simulink subsystem "Controller"  (R2024b)
settings: Solver=VariableStepAuto  StartTime=0.0  StopTime=10.0  RelTol=1e-3
undefined symbols (not defined in the file or in its folder): flight_mode, Parameters, References
libraries: sharedtransform x13, eeGeneralControl x10, simulink x5, aerolibutil x2
(part 2 of 3)

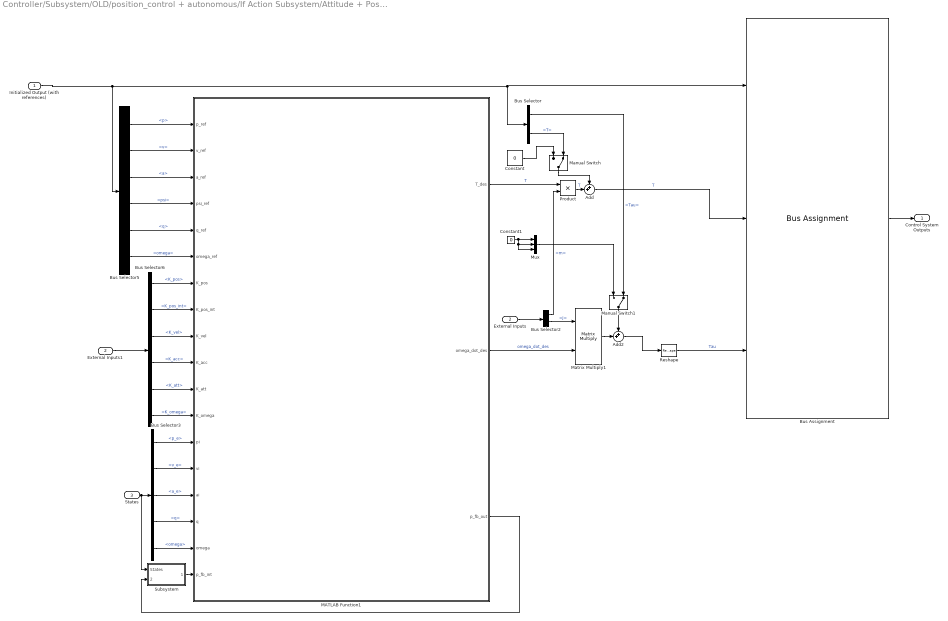
== system Controller/Subsystem/OLD/position_control + autonomous/If Action Subsystem/Attitude + Position FF control1 ==
  Initialized Output (with references) : Inport
  External Inputs : Inport  Port=2
  States : Inport  Port=3
  Add : Sum  Inputs=++|
  Add2 : Sum  Inputs=++|
  Bus Assignment : BusAssignment  AssignedSignals=Control Outputs.T,Control Outputs.Tau
  Bus Selector : BusSelector  OutputSignals=References.reconstructed.Tau,References.reconstructed.T
  Bus Selector2 : BusSelector  OutputSignals=Vehicle Parameters.m,Vehicle Parameters.J
  Bus Selector3 : BusSelector  OutputSignals=p_e,v_e,a_e,q,omega
  Bus Selector5 : BusSelector  OutputSignals=References.trajectory.p,References.trajectory.v,References.trajectory.a,References.trajectory.psi,References.reconstructed.q,References.reconstructed.omega
  Bus Selector6 : BusSelector  OutputSignals=Control Gains.K_pos,Control Gains.K_pos_int,Control Gains.K_vel,Control Gains.K_acc,Control Gains.K_att,Control Gains.K_omega
  Constant : Constant  Value=0
  Constant1 : Constant  Value=0
  External Inputs1 : InportShadow  Port=2
  MATLAB Function1 : MATLAB Function  TreatAsAtomicUnit=on
  Manual Switch : ManualSwitch  CurrentSetting=0
  Manual Switch1 : ManualSwitch  CurrentSetting=0
  Matrix Multiply1 : Product  Multiplication=Matrix(*)
  Mux : Mux  Inputs=3
  Product : Product
  Reshape : Reshape  OutputDimensionality=Column vector (2-D)
  Subsystem : Subsystem
  Control System Outputs : Outport
  wires:
  Manual Switch1/1 -> Add2/1
  Mux/1 -> Manual Switch1/1
  Constant1/1 -> Mux/1, Mux/2, Mux/3
  Constant/1 -> Manual Switch/1
  Manual Switch/1 -> Add/1
  Subsystem/1(p_fb_int) -> MATLAB Function1/18(p_fb_int)
  MATLAB Function1/3(p_fb_out) -> Subsystem/2(p_fb_out)
  Bus Selector6/2 -> MATLAB Function1/8(K_pos_int)  "<K_pos_int>"
  MATLAB Function1/2(omega_dot_des) -> Matrix Multiply1/2  "omega_dot_des"
  Bus Selector6/6 -> MATLAB Function1/12(K_omega)  "<K_omega>"
  Bus Selector6/5 -> MATLAB Function1/11(K_att)  "<K_att>"
  Initialized Output (with references)/1 -> Bus Assignment/1, Bus Selector/1, Bus Selector5/1
  Bus Selector5/4 -> MATLAB Function1/4(psi_ref)  "<psi>"
  Bus Selector6/4 -> MATLAB Function1/10(K_acc)  "<K_acc>"
  Bus Selector6/3 -> MATLAB Function1/9(K_vel)  "<K_vel>"
  Bus Selector6/1 -> MATLAB Function1/7(K_pos)  "<K_pos>"
  External Inputs1/1 -> Bus Selector6/1
  Bus Selector2/2 -> Matrix Multiply1/1  "<J>"
  External Inputs/1 -> Bus Selector2/1
  Matrix Multiply1/1 -> Add2/2
  Add2/1 -> Reshape/1
  Bus Selector/1 -> Manual Switch1/2  "<Tau>"
  Bus Selector/2 -> Manual Switch/2  "<T>"
  Bus Selector3/3 -> MATLAB Function1/15(ai)  "<a_e>"
  Bus Selector3/2 -> MATLAB Function1/14(vi)  "<v_e>"
  Bus Selector3/5 -> MATLAB Function1/17(omega)  "<omega>"
  Bus Selector3/4 -> MATLAB Function1/16(q)  "<q>"
  Bus Selector3/1 -> MATLAB Function1/13(pi)  "<p_e>"
  States/1 -> Bus Selector3/1, Subsystem/1(States)
  Bus Selector5/6 -> MATLAB Function1/6(omega_ref)  "<omega>"
  Bus Selector5/5 -> MATLAB Function1/5(q_ref)  "<q>"
  Bus Selector5/3 -> MATLAB Function1/3(a_ref)  "<a>"
  Bus Selector5/2 -> MATLAB Function1/2(v_ref)  "<v>"
  Bus Selector5/1 -> MATLAB Function1/1(p_ref)  "<p>"
  Bus Assignment/1 -> Control System Outputs/1
  Reshape/1 -> Bus Assignment/3  "Tau"
  Add/1 -> Bus Assignment/2  "T"
  Bus Selector2/1 -> Product/2  "<m>"
  MATLAB Function1/1(T_des) -> Product/1  "T"
  Product/1 -> Add/2  "T"

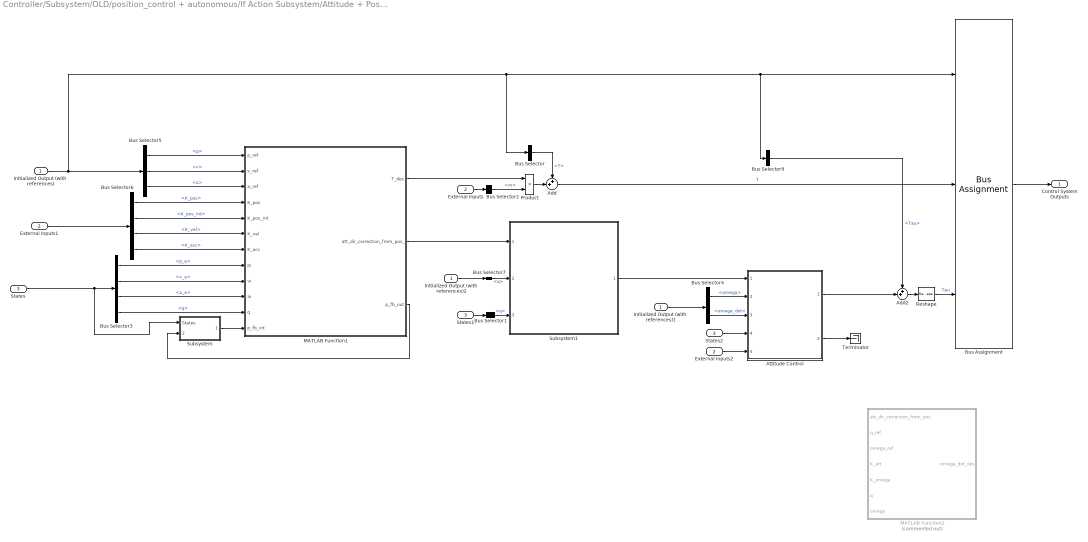
== system Controller/Subsystem/OLD/position_control + autonomous/If Action Subsystem/Attitude + Position FF control2 ==
  Initialized Output (with references) : Inport
  External Inputs : Inport  Port=2
  States : Inport  Port=3
  Add : Sum  Inputs=++|
  Add2 : Sum  Inputs=++|
  Attitude Control : Subsystem  ReferencedSubsystem=Attitude_Control
  Bus Assignment : BusAssignment  AssignedSignals=Control Outputs.T,Control Outputs.Tau
  Bus Selector : BusSelector  OutputSignals=References.reconstructed.T
  Bus Selector1 : BusSelector  OutputSignals=q
  Bus Selector2 : BusSelector  OutputSignals=Vehicle Parameters.m
  Bus Selector3 : BusSelector  OutputSignals=p_e,v_e,a_e,q
  Bus Selector4 : BusSelector  OutputSignals=References.reconstructed.omega,References.reconstructed.omega_dot
  Bus Selector5 : BusSelector  OutputSignals=References.trajectory.p,References.trajectory.v,References.trajectory.a
  Bus Selector6 : BusSelector  OutputSignals=Control Gains.K_pos,Control Gains.K_pos_int,Control Gains.K_vel,Control Gains.K_acc
  Bus Selector7 : BusSelector  OutputSignals=References.reconstructed.q
  Bus Selector9 : BusSelector  OutputSignals=References.reconstructed.Tau
  External Inputs1 : InportShadow  Port=2
  External Inputs2 : InportShadow  Port=2
  Initialized Output (with references)1 : InportShadow
  Initialized Output (with references)2 : InportShadow
  MATLAB Function1 : MATLAB Function  TreatAsAtomicUnit=on
  MATLAB Function2 : MATLAB Function  Commented=on  TreatAsAtomicUnit=on
  Product : Product
  Reshape : Reshape  OutputDimensionality=Column vector (2-D)
  States1 : InportShadow  Port=3
  States2 : InportShadow  Port=3
  Subsystem : Subsystem
  Subsystem1 : Subsystem  ReferencedSubsystem=CombineOuterLoopFB_with_FF_att_ref
  Terminator : Terminator
  Control System Outputs : Outport
  wires:
  Bus Selector9/1 -> Add2/1  "<Tau>"
  Subsystem/1(p_fb_int) -> MATLAB Function1/12(p_fb_int)
  MATLAB Function1/3(p_fb_out) -> Subsystem/2(p_fb_out)
  Bus Selector6/2 -> MATLAB Function1/5(K_pos_int)  "<K_pos_int>"
  Bus Selector6/4 -> MATLAB Function1/7(K_acc)  "<K_acc>"
  Bus Selector6/3 -> MATLAB Function1/6(K_vel)  "<K_vel>"
  Bus Selector6/1 -> MATLAB Function1/4(K_pos)  "<K_pos>"
  Attitude Control/1 -> Add2/2
  Add2/1 -> Reshape/1
  Bus Selector/1 -> Add/1  "<T>"
  Bus Selector3/3 -> MATLAB Function1/10(ai)  "<a_e>"
  Bus Selector3/2 -> MATLAB Function1/9(vi)  "<v_e>"
  Bus Selector3/4 -> MATLAB Function1/11(q)  "<q>"
  Bus Selector3/1 -> MATLAB Function1/8(pi)  "<p_e>"
  Bus Selector5/3 -> MATLAB Function1/3(a_ref)  "<a>"
  Bus Selector5/2 -> MATLAB Function1/2(v_ref)  "<v>"
  Bus Selector5/1 -> MATLAB Function1/1(p_ref)  "<p>"
  Bus Assignment/1 -> Control System Outputs/1
  Reshape/1 -> Bus Assignment/3  "Tau"
  Add/1 -> Bus Assignment/2  "T"
  Bus Selector2/1 -> Product/2  "<m>"
  Bus Selector4/1 -> Attitude Control/2  "<omega>"
  Initialized Output (with references)/1 -> Bus Selector5/1, Bus Selector/1, Bus Selector9/1, Bus Assignment/1
  External Inputs1/1 -> Bus Selector6/1
  States/1 -> Subsystem/1(States), Bus Selector3/1
  Product/1 -> Add/2
  MATLAB Function1/2(att_dir_correction_from_pos_) -> Subsystem1/1
  MATLAB Function1/1(T_des) -> Product/1
  External Inputs/1 -> Bus Selector2/1
  Initialized Output (with references)1/1 -> Bus Selector4/1
  Bus Selector4/2 -> Attitude Control/3  "<omega_dot>"
  Attitude Control/2 -> Terminator/1
  Subsystem1/1 -> Attitude Control/1
  External Inputs2/1 -> Attitude Control/5
  States2/1 -> Attitude Control/4
  Initialized Output (with references)2/1 -> Bus Selector7/1
  States1/1 -> Bus Selector1/1
  Bus Selector1/1 -> Subsystem1/3  "<q>"
  Bus Selector7/1 -> Subsystem1/2  "<q>"

== system Controller/Subsystem/OLD/position_control + autonomous/K-matrix control/K-matrix-control ==
  Initialized Output (with references) : Inport
  External Inputs : Inport  Port=2
  States : Inport  Port=3
  Bus Assignment : BusAssignment  AssignedSignals=Control Outputs.Tau,Control Outputs.T
  Bus Selector : BusSelector  OutputSignals=References.trajectory.p,References.trajectory.v,References.reconstructed.q,References.reconstructed.omega,References.reconstructed.T,References.reconstructed.Tau
  Bus Selector1 : BusSelector  OutputSignals=Control Gains.K_matrix_control.K_pos_int
  Bus Selector3 : BusSelector  OutputSignals=p_e,v_e,q,omega_b
  Bus Selector4 : BusSelector  OutputSignals=Control Gains.K_matrix_control.K
  External Inputs1 : InportShadow  Port=2
  MATLAB Function2 : MATLAB Function  TreatAsAtomicUnit=on
  Product : Product  Multiplication=Matrix(*)
  Reshape : Reshape  OutputDimensionality=Column vector (2-D)
  States1 : InportShadow  Port=3
  Subsystem : Subsystem
  Subsystem3 : Subsystem
  Control System Outputs : Outport
  wires:
  Subsystem/1(att) -> MATLAB Function2/8(att_ref)
  Bus Selector/3 -> Subsystem/1(q)  "<q>"
  Bus Selector/4 -> MATLAB Function2/9(w_ref)  "<omega>"
  Bus Selector/5 -> MATLAB Function2/10(T_ref)  "<T>"
  Bus Selector/6 -> MATLAB Function2/11(Tau_ref)  "<Tau>"
  Bus Selector4/1 -> MATLAB Function2/5(K)  "<K>"
  States/1 -> Bus Selector3/1
  Bus Selector3/4 -> MATLAB Function2/4(omega)  "<omega_b>"
  Bus Selector3/3 -> MATLAB Function2/3(q)  "<q>"
  External Inputs/1 -> Bus Selector4/1
  MATLAB Function2/2(T_des) -> Bus Assignment/3  "T"
  Reshape/1 -> Bus Assignment/2  "Tau"
  MATLAB Function2/1(Tau_des) -> Reshape/1
  Initialized Output (with references)/1 -> Bus Assignment/1, Bus Selector/1
  Bus Assignment/1 -> Control System Outputs/1
  States1/1 -> Subsystem3/1(States)
  Subsystem3/1(p_fb_int) -> Product/2
  MATLAB Function2/3(p_fb_out) -> Subsystem3/2(p_fb_out)
  External Inputs1/1 -> Bus Selector1/1
  Bus Selector1/1 -> Product/1  "<K_pos_int>"
  Bus Selector/2 -> MATLAB Function2/7(V_ref)  "<v>"
  Bus Selector/1 -> MATLAB Function2/6(R_ref)  "<p>"
  Bus Selector3/1 -> MATLAB Function2/1(pi)  "<p_e>"
  Bus Selector3/2 -> MATLAB Function2/2(vi)  "<v_e>"
  Product/1 -> MATLAB Function2/12(p_fb_int)

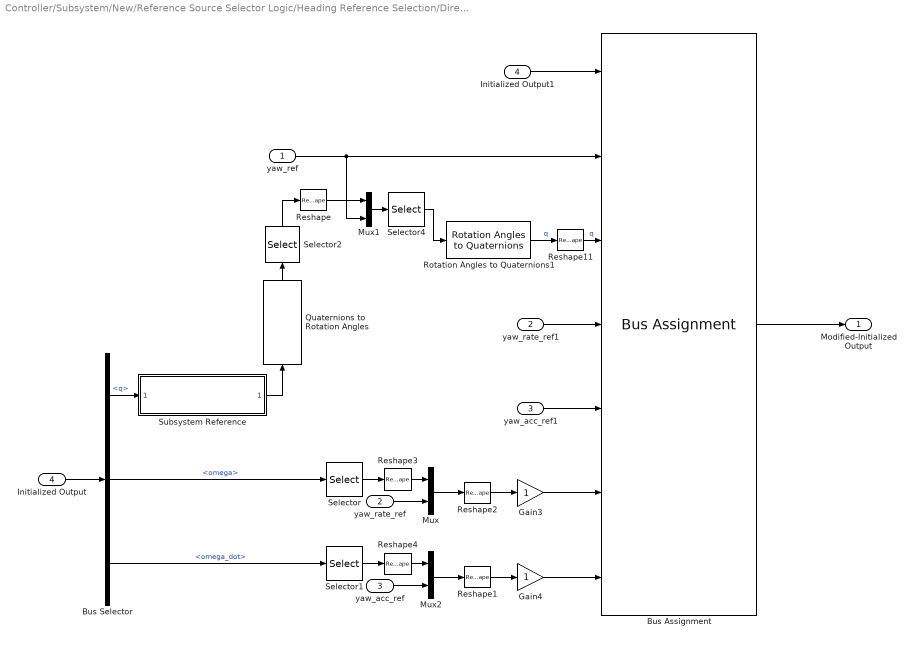
== system Controller/Subsystem/New/Reference Source Selector Logic/Heading Reference Selection/Direct Yaw Command/Subsystem ==
  yaw_ref : Inport
  yaw_rate_ref : Inport  Port=2
  yaw_acc_ref : Inport  Port=3
  Initialized Output : Inport  Port=4
  Bus Assignment : BusAssignment  AssignedSignals=References.trajectory.psi,References.reconstructed.q,References.trajectory.psi_dot,References.trajectory.psi_ddot,References.reconstructed.omega,References.reconstructed.omega_dot
  Bus Selector : BusSelector  OutputSignals=References.reconstructed.q,References.reconstructed.omega,References.reconstructed.omega_dot
  Gain3 : Gain
  Gain4 : Gain
  Initialized Output1 : InportShadow  Port=4
  Mux : Mux  Inputs=2
  Mux1 : Mux  Inputs=2
  Mux2 : Mux  Inputs=2
  Quaternions to Rotation Angles : sharedtransform/Quaternions to Rotation Angles  rotationOrder=ZYX  aMode=aMode
  Reshape : Reshape
  Reshape1 : Reshape  OutputDimensionality=Column vector (2-D)
  Reshape11 : Reshape  OutputDimensionality=Row vector (2-D)
  Reshape2 : Reshape  OutputDimensionality=Column vector (2-D)
  Reshape3 : Reshape
  Reshape4 : Reshape
  Rotation Angles to Quaternions1 : sharedtransform/Rotation Angles to Quaternions  rotationOrder=ZYX  aMode=aMode
  Selector : Selector  InputPortWidth=3  IndexOptions=Index vector (dialog)  Indices=[1 2]  OutputSizes=1
  Selector1 : Selector  InputPortWidth=3  IndexOptions=Index vector (dialog)  Indices=[1 2]  OutputSizes=1
  Selector2 : Selector  InputPortWidth=3  IndexOptions=Index vector (dialog)  Indices=[3 2]  OutputSizes=1
  Selector4 : Selector  InputPortWidth=3  IndexOptions=Index vector (dialog)  Indices=[3 2 1]  OutputSizes=1
  Subsystem Reference : Subsystem  ReferencedSubsystem=Check_Quat
  yaw_acc_ref1 : InportShadow  Port=3
  yaw_rate_ref1 : InportShadow  Port=2
  Modified-Initialized Output : Outport
  wires:
  Bus Assignment/1 -> Modified-Initialized Output/1
  yaw_acc_ref/1 -> Mux2/2
  Gain4/1 -> Bus Assignment/7
  Gain3/1 -> Bus Assignment/6
  yaw_rate_ref/1 -> Mux/2
  Reshape1/1 -> Gain4/1
  Reshape2/1 -> Gain3/1
  Bus Selector/3 -> Selector1/1  "<omega_dot>"
  Selector/1 -> Reshape3/1
  Reshape3/1 -> Mux/1
  Mux/1 -> Reshape2/1
  Selector1/1 -> Reshape4/1
  Reshape4/1 -> Mux2/1
  Mux2/1 -> Reshape1/1
  Initialized Output/1 -> Bus Selector/1
  Bus Selector/2 -> Selector/1  "<omega>"
  Bus Selector/1 -> Subsystem Reference/1  "<q>"
  yaw_ref/1 -> Mux1/2, Bus Assignment/2
  Quaternions to Rotation Angles/1 -> Selector2/1
  Selector2/1 -> Reshape/1
  Reshape/1 -> Mux1/1
  Rotation Angles to Quaternions1/1 -> Reshape11/1  "q"
  Reshape11/1 -> Bus Assignment/3  "q"
  Mux1/1 -> Selector4/1
  Selector4/1 -> Rotation Angles to Quaternions1/1
  yaw_rate_ref1/1 -> Bus Assignment/4
  yaw_acc_ref1/1 -> Bus Assignment/5
  Initialized Output1/1 -> Bus Assignment/1
  Subsystem Reference/1 -> Quaternions to Rotation Angles/1

== system Controller/Subsystem/New/Reference Source Selector Logic/Thrust Reference Selection/Direct Thrust Command/Subsystem1 ==
  T : Inport
  Initialized Output : Inport  Port=2
  Bus Assignment : BusAssignment  AssignedSignals=References.reconstructed.T,Control Outputs.T
  Control Outputs : Outport
  wires:
  Bus Assignment/1 -> Control Outputs/1
  Initialized Output/1 -> Bus Assignment/1
  T/1 -> Bus Assignment/3, Bus Assignment/2  "T"

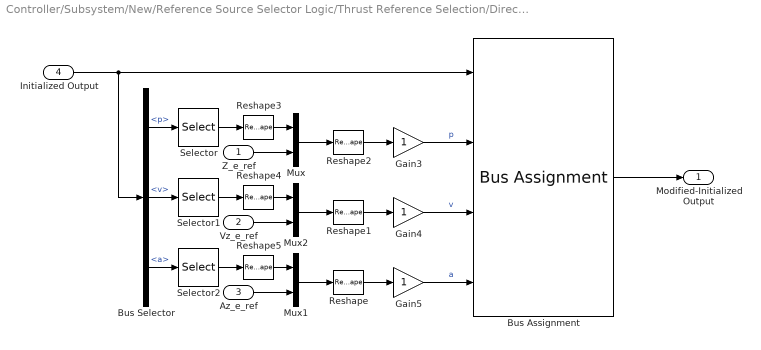
== system Controller/Subsystem/New/Reference Source Selector Logic/Thrust Reference Selection/Direct Z Position Command/Subsystem ==
  Z_e_ref : Inport
  Vz_e_ref : Inport  Port=2
  Az_e_ref : Inport  Port=3
  Initialized Output : Inport  Port=4
  Bus Assignment : BusAssignment  AssignedSignals=References.trajectory.p,References.trajectory.v,References.trajectory.a
  Bus Selector : BusSelector  OutputSignals=References.trajectory.p,References.trajectory.v,References.trajectory.a
  Gain3 : Gain
  Gain4 : Gain
  Gain5 : Gain
  Mux : Mux  Inputs=2
  Mux1 : Mux  Inputs=2
  Mux2 : Mux  Inputs=2
  Reshape : Reshape  OutputDimensionality=Column vector (2-D)
  Reshape1 : Reshape  OutputDimensionality=Column vector (2-D)
  Reshape2 : Reshape  OutputDimensionality=Column vector (2-D)
  Reshape3 : Reshape
  Reshape4 : Reshape
  Reshape5 : Reshape
  Selector : Selector  InputPortWidth=3  IndexOptions=Index vector (dialog)  Indices=[1 2]  OutputSizes=1
  Selector1 : Selector  InputPortWidth=3  IndexOptions=Index vector (dialog)  Indices=[1 2]  OutputSizes=1
  Selector2 : Selector  InputPortWidth=3  IndexOptions=Index vector (dialog)  Indices=[1 2]  OutputSizes=1
  Modified-Initialized Output : Outport
  wires:
  Bus Assignment/1 -> Modified-Initialized Output/1
  Vz_e_ref/1 -> Mux2/2
  Gain4/1 -> Bus Assignment/3  "v"
  Gain5/1 -> Bus Assignment/4  "a"
  Gain3/1 -> Bus Assignment/2  "p"
  Z_e_ref/1 -> Mux/2
  Reshape/1 -> Gain5/1
  Reshape1/1 -> Gain4/1
  Reshape2/1 -> Gain3/1
  Bus Selector/1 -> Selector/1  "<p>"
  Bus Selector/2 -> Selector1/1  "<v>"
  Bus Selector/3 -> Selector2/1  "<a>"
  Selector/1 -> Reshape3/1
  Reshape3/1 -> Mux/1
  Mux/1 -> Reshape2/1
  Selector1/1 -> Reshape4/1
  Reshape4/1 -> Mux2/1
  Mux2/1 -> Reshape1/1
  Mux1/1 -> Reshape/1
  Reshape5/1 -> Mux1/1
  Selector2/1 -> Reshape5/1
  Az_e_ref/1 -> Mux1/2
  Initialized Output/1 -> Bus Selector/1, Bus Assignment/1

== system Controller/Subsystem/New/Reference Source Selector Logic/[X, Y] and//or [Roll, Pitch] Reference Selection/Direct Roll and Pitch Command/Subsystem1 ==
  Roll_Pitch_ref : Inport
  Roll_Pitch_Rate_ref : Inport  Port=2
  Roll_Pitch_Acc_ref : Inport  Port=3
  Initialized Output : Inport  Port=4
  Bus Assignment : BusAssignment  AssignedSignals=References.reconstructed.q,References.reconstructed.omega,References.reconstructed.omega_dot
  Bus Selector : BusSelector  OutputSignals=References.trajectory.psi,References.trajectory.psi_dot,References.trajectory.psi_ddot
  Mux : Mux  Inputs=2
  Mux1 : Mux  Inputs=2
  Mux2 : Mux  Inputs=2
  Reshape : Reshape
  Reshape1 : Reshape
  Reshape11 : Reshape  OutputDimensionality=Row vector (2-D)
  Reshape2 : Reshape
  Reshape7 : Reshape  OutputDimensionality=Column vector (2-D)
  Reshape8 : Reshape  OutputDimensionality=Column vector (2-D)
  Rotation Angles to Quaternions : sharedtransform/Rotation Angles to Quaternions  rotationOrder=ZYX  aMode=aMode
  Selector2 : Selector  InputPortWidth=3  IndexOptions=Index vector (dialog)  Indices=[3 2 1]  OutputSizes=1
  Control Outputs : Outport
  wires:
  Selector2/1 -> Rotation Angles to Quaternions/1
  Bus Assignment/1 -> Control Outputs/1
  Initialized Output/1 -> Bus Selector/1, Bus Assignment/1
  Mux2/1 -> Reshape8/1
  Reshape11/1 -> Bus Assignment/2  "q"
  Reshape8/1 -> Bus Assignment/4  "omega_dot"
  Rotation Angles to Quaternions/1 -> Reshape11/1  "q"
  Reshape7/1 -> Bus Assignment/3  "omega"
  Mux/1 -> Selector2/1
  Mux1/1 -> Reshape7/1
  Roll_Pitch_ref/1 -> Reshape/1
  Bus Selector/1 -> Mux/2  "<psi>"
  Reshape/1 -> Mux/1
  Roll_Pitch_Rate_ref/1 -> Reshape1/1
  Reshape1/1 -> Mux1/1
  Bus Selector/2 -> Mux1/2  "<psi_dot>"
  Bus Selector/3 -> Mux2/2  "<psi_ddot>"
  Reshape2/1 -> Mux2/1
  Roll_Pitch_Acc_ref/1 -> Reshape2/1

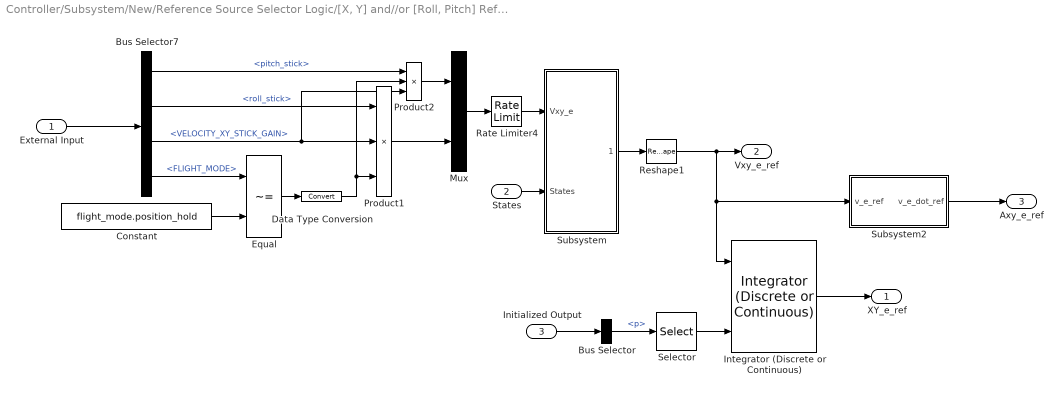
== system Controller/Subsystem/New/Reference Source Selector Logic/[X, Y] and//or [Roll, Pitch] Reference Selection/Direct XY Position Command /Direct XY Position Command  ==
  External Input : Inport
  States : Inport  Port=2
  Initialized Output : Inport  Port=3
  Bus Selector : BusSelector  OutputSignals=References.trajectory.p
  Bus Selector7 : BusSelector  OutputSignals=Pilot Input.Sticks.pitch_stick,Pilot Input.Sticks.roll_stick,Pilot Input.Parameters.VELOCITY_XY_STICK_GAIN,Pilot Input.FLIGHT_MODE
  Constant : Constant  Value=flight_mode.position_hold
  Data Type Conversion : DataTypeConversion  SaturateOnIntegerOverflow=off  RndMeth=Floor
  Equal : RelationalOperator  Operator=~=  OutDataTypeStr=boolean  RndMeth=Simplest  InputSameDT=off
  Integrator (Discrete or Continuous) : eeGeneralControl/Integrator (Discrete or Continuous)  LabelModeActiveChoice=Discrete  ExternalReset=either  LimitType=Anti-windup  B=inf  A=-inf  Ts=-1
      settings: LibrarySourceBlock=|
      | ee_sl_lib/General Control/Integrator
      | (Discrete or Continuous)
  Mux : Mux  Inputs=2
  Product1 : Product  Inputs=3
  Product2 : Product  Inputs=3
  Rate Limiter4 : RateLimiter  RisingSlewLimit=3  FallingSlewLimit=-3  SampleTimeMode=inherited
  Reshape1 : Reshape
  Selector : Selector  InputPortWidth=3  IndexOptions=Index vector (dialog)  Indices=[1 2]  OutputSizes=1
  Subsystem : Subsystem
  Subsystem2 : Subsystem
  XY_e_ref : Outport
  Vxy_e_ref : Outport  Port=2
  Axy_e_ref : Outport  Port=3
  wires:
  Subsystem/1("[Vx Vy]_b") -> Reshape1/1
  States/1 -> Subsystem/2(States)
  Bus Selector7/3 -> Product2/3, Product1/2  "<VELOCITY_XY_STICK_GAIN>"
  Product2/1 -> Mux/1
  Product1/1 -> Mux/2
  External Input/1 -> Bus Selector7/1
  Bus Selector7/1 -> Product2/1  "<pitch_stick>"
  Bus Selector7/2 -> Product1/1  "<roll_stick>"
  Rate Limiter4/1 -> Subsystem/1(Vxy_e)
  Reshape1/1 -> Subsystem2/1(v_e_ref), Integrator (Discrete or Continuous)/1, Vxy_e_ref/1
  Initialized Output/1 -> Bus Selector/1
  Bus Selector/1 -> Selector/1  "<p>"
  Subsystem2/1(v_e_dot_ref) -> Axy_e_ref/1
  Integrator (Discrete or Continuous)/1 -> XY_e_ref/1
  Selector/1 -> Integrator (Discrete or Continuous)/3
  Equal/1 -> Data Type Conversion/1
  Mux/1 -> Rate Limiter4/1
  Data Type Conversion/1 -> Product2/2, Product1/3
  Constant/1 -> Equal/2
  Bus Selector7/4 -> Equal/1  "<FLIGHT_MODE>"

== system Controller/Subsystem/New/Reference Source Selector Logic/[X, Y] and//or [Roll, Pitch] Reference Selection/Direct XY Position Command /Subsystem1 ==
  XY_e_ref : Inport
  Vxy_e_ref : Inport  Port=2
  Axy_e_ref : Inport  Port=3
  Initialized Output : Inport  Port=4
  Bus Assignment : BusAssignment  AssignedSignals=References.trajectory.p,References.trajectory.v,References.trajectory.a
  Bus Selector : BusSelector  OutputSignals=References.trajectory.p,References.trajectory.v,References.trajectory.a
  Mux : Mux  Inputs=2
  Mux1 : Mux  Inputs=2
  Mux2 : Mux  Inputs=2
  Reshape : Reshape
  Reshape1 : Reshape
  Reshape2 : Reshape
  Reshape3 : Reshape  OutputDimensionality=Column vector (2-D)
  Reshape7 : Reshape  OutputDimensionality=Column vector (2-D)
  Reshape8 : Reshape  OutputDimensionality=Column vector (2-D)
  Selector : Selector  InputPortWidth=3  IndexOptions=Index vector (dialog)  Indices=[3]  OutputSizes=1
  Selector1 : Selector  InputPortWidth=3  IndexOptions=Index vector (dialog)  Indices=[3]  OutputSizes=1
  Selector2 : Selector  InputPortWidth=3  IndexOptions=Index vector (dialog)  Indices=[3]  OutputSizes=1
  Control Outputs : Outport
  wires:
  Bus Assignment/1 -> Control Outputs/1
  Initialized Output/1 -> Bus Selector/1, Bus Assignment/1
  Mux2/1 -> Reshape8/1
  Reshape3/1 -> Bus Assignment/2  "p_e"
  Reshape8/1 -> Bus Assignment/4  "a_e"
  Reshape7/1 -> Bus Assignment/3  "v_e"
  Mux/1 -> Reshape3/1
  Mux1/1 -> Reshape7/1
  XY_e_ref/1 -> Reshape/1
  Bus Selector/1 -> Selector2/1  "<p>"
  Reshape/1 -> Mux/1
  Vxy_e_ref/1 -> Reshape1/1
  Reshape1/1 -> Mux1/1
  Bus Selector/2 -> Selector1/1  "<v>"
  Bus Selector/3 -> Selector/1  "<a>"
  Reshape2/1 -> Mux2/1
  Axy_e_ref/1 -> Reshape2/1
  Selector/1 -> Mux2/2
  Selector1/1 -> Mux1/2
  Selector2/1 -> Mux/2

== system Controller/Subsystem/New/Translational Motion Feedback Selector/Switch Case Action Subsystem/Translational Motion Control/Subsystem ==
  <MIN_TH> : Inport
  <MAX_TH> : Inport  Port=2
  <MAX_THRUST> : Inport  Port=3
  Gain : Gain  Gain=4
  Product : Product
  Product1 : Product
  MIN_TH : Outport
  MAX_TH : Outport  Port=2
  wires:
  Gain/1 -> Product/1, Product1/2
  <MAX_TH>/1 -> Product1/1
  <MIN_TH>/1 -> Product/2
  Product/1 -> MIN_TH/1
  Product1/1 -> MAX_TH/1
  <MAX_THRUST>/1 -> Gain/1

== system Controller/Subsystem/OLD/position_control + autonomous/Guidance/Trajectory Solution Evaluator/Hold current position ==
  Initialized Output : Inport
  Action Port : ActionPort  InitializeStates=reset
  Subsystem1 : Subsystem
  Modified-Initialized Output : Outport
  wires:
  Initialized Output/1 -> Subsystem1/1(Initialized Output)
  Subsystem1/1(Modified-Initialized Output) -> Modified-Initialized Output/1

== system Controller/Subsystem/OLD/position_control + autonomous/Guidance/Trajectory Solution Evaluator/Switch Case Action Subsystem ==
  external_input : Inport
  States : Inport  Port=2
  Initialized Output : Inport  Port=3
  Action Port : ActionPort  InitializeStates=reset
  FF reconstructor : Subsystem  ReferencedSubsystem=FF_reconstructor
  Modified-Initialized Output : Outport
  wires:
  external_input/1 -> FF reconstructor/2
  States/1 -> FF reconstructor/3
  FF reconstructor/1 -> Modified-Initialized Output/1
  Initialized Output/1 -> FF reconstructor/1

== system Controller/Subsystem/OLD/position_control + autonomous/Guidance/Trajectory Solution Evaluator/Switch Case Action Subsystem1 ==
  States : Inport
  external_input : Inport  Port=2
  Initialized Output : Inport  Port=3
  Action Port : ActionPort  InitializeStates=reset
  Constant : Constant  Value=false
  Delay : Delay  DelayLength=1  InitialCondition=true
  Map User Input : Subsystem
  Modified-Initialized Output : Outport
  wires:
  Delay/1 -> Map User Input/4(reset)
  Constant/1 -> Delay/1
  Initialized Output/1 -> Map User Input/3(Initialized Output)
  Map User Input/1(Modified-Initialized Output) -> Modified-Initialized Output/1
  external_input/1 -> Map User Input/1(External Input)
  States/1 -> Map User Input/2(States)

== system Controller/Subsystem/OLD/position_control + autonomous/If Action Subsystem/Attitude + Position FF control/Subsystem ==
  States : Inport
  p_fb_out : Inport  Port=2
  Bus Selector1 : BusSelector  OutputSignals=GC
  If : If  IfExpression=u1
  If Action Subsystem : Subsystem  TreatAsAtomicUnit=on
  If Action Subsystem1 : Subsystem  TreatAsAtomicUnit=on
  Merge : Merge
  p_fb_int : Outport
  wires:
  Merge/1 -> p_fb_int/1
  If Action Subsystem1/1(Out1) -> Merge/2
  If Action Subsystem/1(p_fb_int) -> Merge/1
  If/2 -> If Action Subsystem/Action
  States/1 -> Bus Selector1/1
  p_fb_out/1 -> If Action Subsystem/1(p_fb_out)
  If/1 -> If Action Subsystem1/Action
  Bus Selector1/1 -> If/1  "<GC>"

== system Controller/Subsystem/OLD/position_control + autonomous/If Action Subsystem/Attitude + Position FF control1/Subsystem ==
  States : Inport
  p_fb_out : Inport  Port=2
  Bus Selector1 : BusSelector  OutputSignals=GC
  If : If  IfExpression=u1
  If Action Subsystem : Subsystem  TreatAsAtomicUnit=on
  If Action Subsystem1 : Subsystem  TreatAsAtomicUnit=on
  Merge : Merge
  p_fb_int : Outport
  wires:
  Merge/1 -> p_fb_int/1
  If Action Subsystem1/1(Out1) -> Merge/2
  If Action Subsystem/1(p_fb_int) -> Merge/1
  If/2 -> If Action Subsystem/Action
  States/1 -> Bus Selector1/1
  p_fb_out/1 -> If Action Subsystem/1(p_fb_out)
  If/1 -> If Action Subsystem1/Action
  Bus Selector1/1 -> If/1  "<GC>"

== system Controller/Subsystem/OLD/position_control + autonomous/If Action Subsystem/Attitude + Position FF control2/Subsystem ==
  States : Inport
  p_fb_out : Inport  Port=2
  Bus Selector1 : BusSelector  OutputSignals=GC
  If : If  IfExpression=u1
  If Action Subsystem : Subsystem  TreatAsAtomicUnit=on
  If Action Subsystem1 : Subsystem  TreatAsAtomicUnit=on
  Merge : Merge
  p_fb_int : Outport
  wires:
  Merge/1 -> p_fb_int/1
  If Action Subsystem1/1(Out1) -> Merge/2
  If Action Subsystem/1(p_fb_int) -> Merge/1
  If/2 -> If Action Subsystem/Action
  States/1 -> Bus Selector1/1
  p_fb_out/1 -> If Action Subsystem/1(p_fb_out)
  If/1 -> If Action Subsystem1/Action
  Bus Selector1/1 -> If/1  "<GC>"

== system Controller/Subsystem/OLD/position_control + autonomous/K-matrix control/K-matrix-control/Subsystem ==
  q : Inport
  Quaternions to Rotation Angles : sharedtransform/Quaternions to Rotation Angles  rotationOrder=ZYX  aMode=aMode
  Reshape1 : Reshape  OutputDimensionality=Column vector (2-D)
  Selector : Selector  InputPortWidth=3  IndexOptions=Index vector (dialog)  Indices=[3 2 1]  OutputSizes=1
  att : Outport
  wires:
  Reshape1/1 -> att/1
  q/1 -> Quaternions to Rotation Angles/1
  Quaternions to Rotation Angles/1 -> Selector/1
  Selector/1 -> Reshape1/1

== system Controller/Subsystem/OLD/position_control + autonomous/K-matrix control/K-matrix-control/Subsystem3 ==
  States : Inport
  p_fb_out : Inport  Port=2
  Bus Selector1 : BusSelector  OutputSignals=GC
  If : If  IfExpression=u1
  If Action Subsystem : Subsystem  TreatAsAtomicUnit=on
  If Action Subsystem1 : Subsystem  TreatAsAtomicUnit=on
  Merge : Merge
  p_fb_int : Outport
  wires:
  Merge/1 -> p_fb_int/1
  If Action Subsystem1/1(Out1) -> Merge/2
  If Action Subsystem/1(p_fb_int) -> Merge/1
  If/2 -> If Action Subsystem/Action
  States/1 -> Bus Selector1/1
  p_fb_out/1 -> If Action Subsystem/1(p_fb_out)
  If/1 -> If Action Subsystem1/Action
  Bus Selector1/1 -> If/1  "<GC>"

== system Controller/Subsystem/New/Reference Source Selector Logic/[X, Y] and//or [Roll, Pitch] Reference Selection/Direct XY Position Command /Direct XY Position Command /Subsystem ==
  Vxy_e : Inport
  States : Inport  Port=2
  Bus Selector1 : BusSelector  OutputSignals=att
  Constant : Constant  Value=0
  Gain : Gain  Gain=-1
  Mux1 : Mux  Inputs=3
  Mux2 : Mux  Inputs=2
  Quaternion Rotation : aerolibutil/Quaternion Rotation
  Rotation Angles to Quaternions : sharedtransform/Rotation Angles to Quaternions  rotationOrder=ZYX  aMode=aMode
  Selector : Selector  InputPortWidth=3  IndexOptions=Index vector (dialog)  Indices=[3]  OutputSizes=1
  Selector1 : Selector  InputPortWidth=3  IndexOptions=Index vector (dialog)  Indices=[1,2]  OutputSizes=1
  "[Vx Vy]_b" : Outport
  wires:
  Gain/1 -> Mux1/1
  Vxy_e/1 -> Mux2/1
  Rotation Angles to Quaternions/1 -> Quaternion Rotation/1
  Bus Selector1/1 -> Selector/1  "<att>"
  Selector/1 -> Gain/1
  Quaternion Rotation/1 -> Selector1/1
  Constant/1 -> Mux1/2, Mux2/2, Mux1/3
  Mux2/1 -> Quaternion Rotation/2
  States/1 -> Bus Selector1/1
  Mux1/1 -> Rotation Angles to Quaternions/1
  Selector1/1 -> "[Vx Vy]_b"/1

== system Controller/Subsystem/New/Reference Source Selector Logic/[X, Y] and//or [Roll, Pitch] Reference Selection/Direct XY Position Command /Direct XY Position Command /Subsystem2 ==
  v_e_ref : Inport
  Discrete Derivative : simulink/Discrete/Discrete Derivative  gainval=1.0  ICPrevScaledInput=0.0  OutMin=[]  OutMax=[]  OutDataType=fixdt(1, 16)  OutScaling=2^-10  DoSatur=off
  Low-Pass Filter (Discrete or Continuous) : eeGeneralControl/Low-Pass Filter (Discrete or Continuous)  K=1  T=1/40  B=inf  A=-inf  init_option=Inherited from block input  x0=0  Ts=-1
  v_e_dot_ref : Outport
  wires:
  Low-Pass Filter (Discrete or Continuous)/1 -> v_e_dot_ref/1
  v_e_ref/1 -> Discrete Derivative/1
  Discrete Derivative/1 -> Low-Pass Filter (Discrete or Continuous)/1

== system Controller/Subsystem/OLD/position_control + autonomous/Guidance/Trajectory Solution Evaluator/Hold current position/Subsystem1 ==
  Initialized Output : Inport
  Bus Selector : BusSelector  OutputSignals=References.trajectory.psi
  Constant : Constant  Value=zeros(3,1)
  Constant1 : Constant  Value=0
  Mux1 : Mux  Inputs=3
  Subsystem : Subsystem
  Modified-Initialized Output : Outport
  wires:
  Mux1/1 -> Subsystem/3(att_ref)
  Constant1/1 -> Mux1/2, Mux1/1
  Bus Selector/1 -> Mux1/3  "<psi>"
  Initialized Output/1 -> Bus Selector/1, Subsystem/6(Initialized Output)
  Constant/1 -> Subsystem/2(a_e_ref), Subsystem/1(v_e_ref), Subsystem/4(omega_ref), Subsystem/5(omega_dot)
  Subsystem/1(Modified-Initialized Output) -> Modified-Initialized Output/1

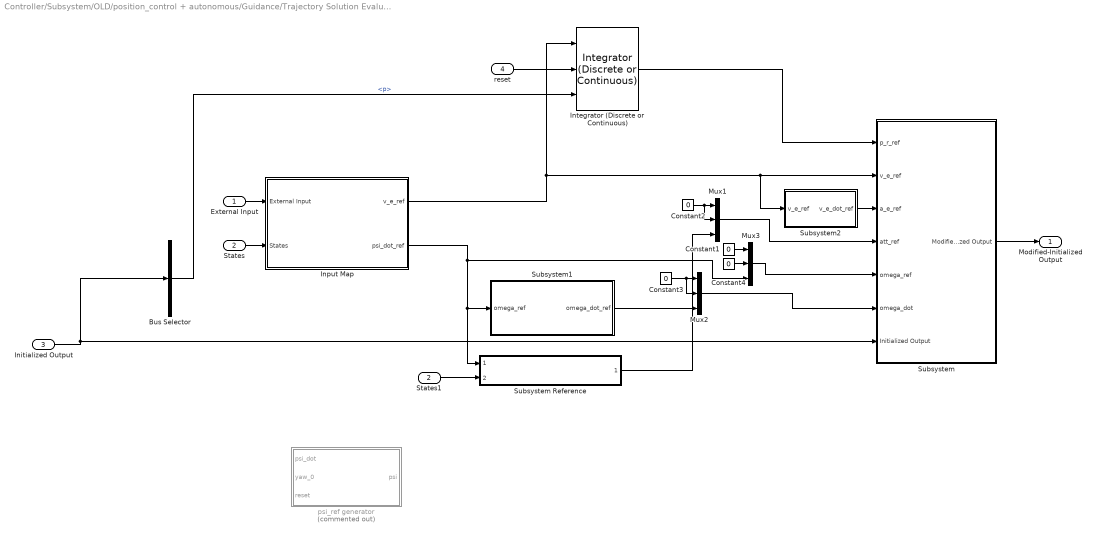
== system Controller/Subsystem/OLD/position_control + autonomous/Guidance/Trajectory Solution Evaluator/Switch Case Action Subsystem1/Map User Input ==
  External Input : Inport
  States : Inport  Port=2
  Initialized Output : Inport  Port=3
  reset : Inport  Port=4
  Bus Selector : BusSelector  OutputSignals=References.trajectory.p
  Constant{1..4} (4 alike) : Constant  Value=0
  Input Map : Subsystem
  Integrator (Discrete or Continuous) : eeGeneralControl/Integrator (Discrete or Continuous)  LabelModeActiveChoice=Discrete  ExternalReset=rising  LimitType=Anti-windup  B=inf  A=-inf  Ts=-1
      settings: LibrarySourceBlock=|
      | ee_sl_lib/General Control/Integrator
      | (Discrete or Continuous)
  Mux1 : Mux  Inputs=3
  Mux2 : Mux  Inputs=3
  Mux3 : Mux  Inputs=3
  States1 : InportShadow  Port=2
  Subsystem : Subsystem
  Subsystem Reference : Subsystem  ReferencedSubsystem=heading_generator
  Subsystem1 : Subsystem
  Subsystem2 : Subsystem
  psi_ref generator : Subsystem  Commented=on
  Modified-Initialized Output : Outport
  wires:
  reset/1 -> Integrator (Discrete or Continuous)/2
  Bus Selector/1 -> Integrator (Discrete or Continuous)/3  "<p>"
  Constant3/1 -> Mux2/2, Mux2/1
  Mux2/1 -> Subsystem/6(omega_dot)
  Input Map/1(v_e_ref) -> Integrator (Discrete or Continuous)/1, Subsystem2/1(v_e_ref), Subsystem/2(v_e_ref)
  Input Map/2(psi_dot_ref) -> Mux3/3, Subsystem Reference/1, Subsystem1/1(omega_ref)
  External Input/1 -> Input Map/1(External Input)
  Integrator (Discrete or Continuous)/1 -> Subsystem/1(p_r_ref)
  Mux1/1 -> Subsystem/4(att_ref)
  Initialized Output/1 -> Subsystem/7(Initialized Output), Bus Selector/1
  Subsystem/1(Modified-Initialized Output) -> Modified-Initialized Output/1
  States/1 -> Input Map/2(States)
  Mux3/1 -> Subsystem/5(omega_ref)
  Constant4/1 -> Mux3/2
  Constant2/1 -> Mux1/2, Mux1/1
  Subsystem Reference/1 -> Mux1/3
  Constant1/1 -> Mux3/1
  Subsystem1/1(omega_dot_ref) -> Mux2/3
  Subsystem2/1(v_e_dot_ref) -> Subsystem/3(a_e_ref)
  States1/1 -> Subsystem Reference/2

== system Controller/Subsystem/OLD/position_control + autonomous/If Action Subsystem/Attitude + Position FF control/Subsystem/If Action Subsystem ==
  p_fb_out : Inport
  Action Port : ActionPort  InitializeStates=reset
  Constant : Constant  Value=zeros(3,1)
  Constant1 : Constant  Value=true
  Integrator (Discrete or Continuous) : eeGeneralControl/Integrator (Discrete or Continuous)  LabelModeActiveChoice=Discrete  ExternalReset=either  LimitType=Anti-windup  B=1  A=-1  Ts=-1
      settings: LibrarySourceBlock=|
      | ee_sl_lib/General Control/Integrator
      | (Discrete or Continuous)
  p_fb_int : Outport
  wires:
  p_fb_out/1 -> Integrator (Discrete or Continuous)/1
  Constant/1 -> Integrator (Discrete or Continuous)/3
  Integrator (Discrete or Continuous)/1 -> p_fb_int/1
  Constant1/1 -> Integrator (Discrete or Continuous)/2

== system Controller/Subsystem/OLD/position_control + autonomous/If Action Subsystem/Attitude + Position FF control/Subsystem/If Action Subsystem1 ==
  Action Port : ActionPort
  Constant : Constant  Value=zeros(3,1)
  Out1 : Outport
  wires:
  Constant/1 -> Out1/1

== system Controller/Subsystem/OLD/position_control + autonomous/If Action Subsystem/Attitude + Position FF control1/Subsystem/If Action Subsystem ==
  p_fb_out : Inport
  Action Port : ActionPort  InitializeStates=reset
  Constant : Constant  Value=zeros(3,1)
  Constant1 : Constant  Value=true
  Integrator (Discrete or Continuous) : eeGeneralControl/Integrator (Discrete or Continuous)  LabelModeActiveChoice=Discrete  ExternalReset=either  LimitType=Anti-windup  B=1  A=-1  Ts=-1
      settings: LibrarySourceBlock=|
      | ee_sl_lib/General Control/Integrator
      | (Discrete or Continuous)
  p_fb_int : Outport
  wires:
  p_fb_out/1 -> Integrator (Discrete or Continuous)/1
  Constant/1 -> Integrator (Discrete or Continuous)/3
  Integrator (Discrete or Continuous)/1 -> p_fb_int/1
  Constant1/1 -> Integrator (Discrete or Continuous)/2

== system Controller/Subsystem/OLD/position_control + autonomous/If Action Subsystem/Attitude + Position FF control1/Subsystem/If Action Subsystem1 ==
  Action Port : ActionPort
  Constant : Constant  Value=zeros(3,1)
  Out1 : Outport
  wires:
  Constant/1 -> Out1/1

== system Controller/Subsystem/OLD/position_control + autonomous/If Action Subsystem/Attitude + Position FF control2/Subsystem/If Action Subsystem ==
  p_fb_out : Inport
  Action Port : ActionPort  InitializeStates=reset
  Constant : Constant  Value=zeros(3,1)
  Constant1 : Constant  Value=true
  Integrator (Discrete or Continuous) : eeGeneralControl/Integrator (Discrete or Continuous)  LabelModeActiveChoice=Discrete  ExternalReset=either  LimitType=Anti-windup  B=1  A=-1  Ts=-1
      settings: LibrarySourceBlock=|
      | ee_sl_lib/General Control/Integrator
      | (Discrete or Continuous)
  p_fb_int : Outport
  wires:
  p_fb_out/1 -> Integrator (Discrete or Continuous)/1
  Constant/1 -> Integrator (Discrete or Continuous)/3
  Integrator (Discrete or Continuous)/1 -> p_fb_int/1
  Constant1/1 -> Integrator (Discrete or Continuous)/2

== system Controller/Subsystem/OLD/position_control + autonomous/If Action Subsystem/Attitude + Position FF control2/Subsystem/If Action Subsystem1 ==
  Action Port : ActionPort
  Constant : Constant  Value=zeros(3,1)
  Out1 : Outport
  wires:
  Constant/1 -> Out1/1

== system Controller/Subsystem/OLD/position_control + autonomous/K-matrix control/K-matrix-control/Subsystem3/If Action Subsystem ==
  p_fb_out : Inport
  Action Port : ActionPort  InitializeStates=reset
  Constant : Constant  Value=zeros(6,1)
  Constant1 : Constant  Value=true
  Integrator (Discrete or Continuous) : eeGeneralControl/Integrator (Discrete or Continuous)  LabelModeActiveChoice=Discrete  ExternalReset=either  LimitType=Anti-windup  B=3  A=-3  Ts=-1
      settings: LibrarySourceBlock=|
      | ee_sl_lib/General Control/Integrator
      | (Discrete or Continuous)
  p_fb_int : Outport
  wires:
  p_fb_out/1 -> Integrator (Discrete or Continuous)/1
  Constant/1 -> Integrator (Discrete or Continuous)/3
  Integrator (Discrete or Continuous)/1 -> p_fb_int/1
  Constant1/1 -> Integrator (Discrete or Continuous)/2

== system Controller/Subsystem/OLD/position_control + autonomous/K-matrix control/K-matrix-control/Subsystem3/If Action Subsystem1 ==
  Action Port : ActionPort
  Constant : Constant  Value=zeros(6,1)
  Out1 : Outport
  wires:
  Constant/1 -> Out1/1

== system Controller/Subsystem/OLD/position_control + autonomous/Guidance/Trajectory Solution Evaluator/Hold current position/Subsystem1/Subsystem ==
  v_e_ref : Inport
  a_e_ref : Inport  Port=2
  att_ref : Inport  Port=3
  omega_ref : Inport  Port=4
  omega_dot : Inport  Port=5
  Initialized Output : Inport  Port=6
  Bus Assignment : BusAssignment  AssignedSignals=References.trajectory.v,References.trajectory.a,References.trajectory.psi,References.trajectory.psi_dot,References.reconstructed.q,References.reconstructed.omega,References.reconstructed.omega_dot
  Gain4 : Gain
  Gain5 : Gain
  Reshape{,1,7..8} (4 alike) : Reshape  OutputDimensionality=Column vector (2-D)
  Reshape11 : Reshape  OutputDimensionality=Row vector (2-D)
  Rotation Angles to Quaternions : sharedtransform/Rotation Angles to Quaternions  rotationOrder=ZYX  aMode=aMode
  Selector : Selector  InputPortWidth=3  IndexOptions=Index vector (dialog)  Indices=[3]  OutputSizes=1
  Selector1 : Selector  InputPortWidth=3  IndexOptions=Index vector (dialog)  Indices=[3]  OutputSizes=1
  Selector2 : Selector  InputPortWidth=3  IndexOptions=Index vector (dialog)  Indices=[3,2,1]  OutputSizes=1
  Modified-Initialized Output : Outport
  wires:
  Selector2/1 -> Rotation Angles to Quaternions/1
  Bus Assignment/1 -> Modified-Initialized Output/1
  Initialized Output/1 -> Bus Assignment/1
  omega_dot/1 -> Reshape8/1
  a_e_ref/1 -> Reshape/1
  v_e_ref/1 -> Reshape1/1
  Reshape11/1 -> Bus Assignment/6  "q"
  Reshape8/1 -> Bus Assignment/8  "omega_dot"
  Rotation Angles to Quaternions/1 -> Reshape11/1  "q"
  Reshape7/1 -> Bus Assignment/7  "omega"
  att_ref/1 -> Selector1/1, Selector2/1
  omega_ref/1 -> Reshape7/1, Selector/1
  Selector/1 -> Bus Assignment/5  "psi_dot"
  Gain4/1 -> Bus Assignment/2  "v"
  Selector1/1 -> Bus Assignment/4  "psi"
  Gain5/1 -> Bus Assignment/3  "a"
  Reshape/1 -> Gain5/1
  Reshape1/1 -> Gain4/1

== system Controller/Subsystem/OLD/position_control + autonomous/Guidance/Trajectory Solution Evaluator/Switch Case Action Subsystem1/Map User Input/Input Map ==
  External Input : Inport
  States : Inport  Port=2
  Bus Selector2 : BusSelector  OutputSignals=Pilot Input.Sticks.Throttle_stick,Pilot Input.Parameters.VELOCITY_Z_STICK_GAIN,Pilot Input.Parameters.MANUAL_YAW_RATE_STICK_GAIN,Pilot Input.Parameters.VELOCITY_XY_STICK_GAIN
  Bus Selector7 : BusSelector  OutputSignals=Pilot Input.Sticks.roll_stick,Pilot Input.Sticks.pitch_stick,Pilot Input.Sticks.yaw_stick  OutputAsBus=on
  Demux : Demux  Outputs=3
  Gain : Gain  Gain=-1
  Mux : Mux  Inputs=2
  Product{,1..3} (4 alike) : Product
  Rate Limiter2 : RateLimiter  RisingSlewLimit=0.8  FallingSlewLimit=-0.8  SampleTimeMode=inherited
  Rate Limiter3 : RateLimiter  RisingSlewLimit=3  FallingSlewLimit=-3  SampleTimeMode=inherited
  Rate Limiter4 : RateLimiter  RisingSlewLimit=3  FallingSlewLimit=-3  SampleTimeMode=inherited
  Rate Limiter5 : RateLimiter  RisingSlewLimit=60*pi/180  FallingSlewLimit=-60*pi/180  SampleTimeMode=inherited
  Reshape : Reshape  OutputDimensionality=Column vector (2-D)
  Reshape1 : Reshape
  Subsystem : Subsystem
  v_e_ref : Outport
  psi_dot_ref : Outport  Port=2
  wires:
  Mux/1 -> v_e_ref/1
  Reshape1/1 -> Mux/1
  Subsystem/1("[Vx Vy]_b") -> Reshape1/1
  States/1 -> Subsystem/3(States)
  Rate Limiter2/1 -> Mux/2
  Bus Selector2/4 -> Product1/1, Product2/1  "<VELOCITY_XY_STICK_GAIN>"
  Product2/1 -> Rate Limiter4/1
  Product1/1 -> Rate Limiter3/1
  External Input/1 -> Bus Selector7/1, Bus Selector2/1
  Product/1 -> Rate Limiter2/1
  Demux/2 -> Product2/2
  Bus Selector2/3 -> Product3/1  "<MANUAL_YAW_RATE_STICK_GAIN>"
  Reshape/1 -> Demux/1
  Demux/3 -> Product3/2
  Bus Selector7/1 -> Reshape/1
  Demux/1 -> Product1/2
  Bus Selector2/1 -> Gain/1  "<Throttle_stick>"
  Bus Selector2/2 -> Product/2  "<VELOCITY_Z_STICK_GAIN>"
  Product3/1 -> Rate Limiter5/1
  Gain/1 -> Product/1
  Rate Limiter5/1 -> psi_dot_ref/1
  Rate Limiter3/1 -> Subsystem/1(Vy_e)
  Rate Limiter4/1 -> Subsystem/2(Vx_e)

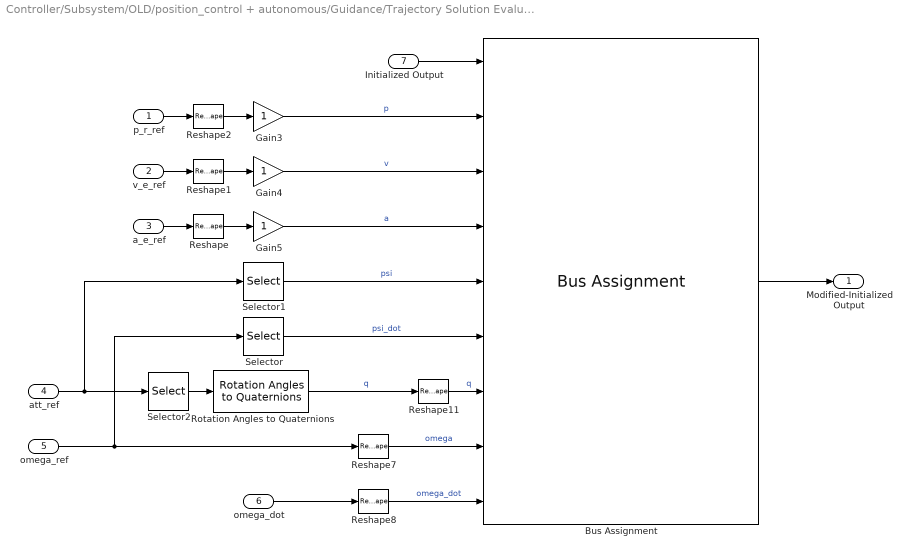
== system Controller/Subsystem/OLD/position_control + autonomous/Guidance/Trajectory Solution Evaluator/Switch Case Action Subsystem1/Map User Input/Subsystem ==
  p_r_ref : Inport
  v_e_ref : Inport  Port=2
  a_e_ref : Inport  Port=3
  att_ref : Inport  Port=4
  omega_ref : Inport  Port=5
  omega_dot : Inport  Port=6
  Initialized Output : Inport  Port=7
  Bus Assignment : BusAssignment  AssignedSignals=References.trajectory.p,References.trajectory.v,References.trajectory.a,References.trajectory.psi,References.trajectory.psi_dot,References.reconstructed.q,References.reconstructed.omega,References.reconstructed.omega_dot
  Gain3 : Gain
  Gain4 : Gain
  Gain5 : Gain
  Reshape{,1..2,7..8} (5 alike) : Reshape  OutputDimensionality=Column vector (2-D)
  Reshape11 : Reshape  OutputDimensionality=Row vector (2-D)
  Rotation Angles to Quaternions : sharedtransform/Rotation Angles to Quaternions  rotationOrder=ZYX  aMode=aMode
  Selector : Selector  InputPortWidth=3  IndexOptions=Index vector (dialog)  Indices=[3]  OutputSizes=1
  Selector1 : Selector  InputPortWidth=3  IndexOptions=Index vector (dialog)  Indices=[3]  OutputSizes=1
  Selector2 : Selector  InputPortWidth=3  IndexOptions=Index vector (dialog)  Indices=[3,2,1]  OutputSizes=1
  Modified-Initialized Output : Outport
  wires:
  Selector2/1 -> Rotation Angles to Quaternions/1
  Bus Assignment/1 -> Modified-Initialized Output/1
  Initialized Output/1 -> Bus Assignment/1
  omega_dot/1 -> Reshape8/1
  a_e_ref/1 -> Reshape/1
  v_e_ref/1 -> Reshape1/1
  Reshape11/1 -> Bus Assignment/7  "q"
  Reshape8/1 -> Bus Assignment/9  "omega_dot"
  Rotation Angles to Quaternions/1 -> Reshape11/1  "q"
  Reshape7/1 -> Bus Assignment/8  "omega"
  att_ref/1 -> Selector1/1, Selector2/1
  omega_ref/1 -> Reshape7/1, Selector/1
  Selector/1 -> Bus Assignment/6  "psi_dot"
  Gain4/1 -> Bus Assignment/3  "v"
  Selector1/1 -> Bus Assignment/5  "psi"
  Gain5/1 -> Bus Assignment/4  "a"
  Gain3/1 -> Bus Assignment/2  "p"
  p_r_ref/1 -> Reshape2/1
  Reshape/1 -> Gain5/1
  Reshape1/1 -> Gain4/1
  Reshape2/1 -> Gain3/1

== system Controller/Subsystem/OLD/position_control + autonomous/Guidance/Trajectory Solution Evaluator/Switch Case Action Subsystem1/Map User Input/Subsystem1 ==
  omega_ref : Inport
  Discrete Derivative : simulink/Discrete/Discrete Derivative  gainval=1.0  ICPrevScaledInput=0.0  OutMin=[]  OutMax=[]  OutDataType=fixdt(1, 16)  OutScaling=2^-10  DoSatur=off
  Low-Pass Filter (Discrete or Continuous) : eeGeneralControl/Low-Pass Filter (Discrete or Continuous)  K=1  T=1/40  B=inf  A=-inf  init_option=Inherited from block input  x0=0  Ts=-1
  omega_dot_ref : Outport
  wires:
  Discrete Derivative/1 -> Low-Pass Filter (Discrete or Continuous)/1
  omega_ref/1 -> Discrete Derivative/1
  Low-Pass Filter (Discrete or Continuous)/1 -> omega_dot_ref/1

== system Controller/Subsystem/OLD/position_control + autonomous/Guidance/Trajectory Solution Evaluator/Switch Case Action Subsystem1/Map User Input/Subsystem2 ==
  v_e_ref : Inport
  Discrete Derivative : simulink/Discrete/Discrete Derivative  gainval=1.0  ICPrevScaledInput=0.0  OutMin=[]  OutMax=[]  OutDataType=fixdt(1, 16)  OutScaling=2^-10  DoSatur=off
  Low-Pass Filter (Discrete or Continuous) : eeGeneralControl/Low-Pass Filter (Discrete or Continuous)  K=1  T=1/40  B=inf  A=-inf  init_option=Inherited from block input  x0=0  Ts=-1
  v_e_dot_ref : Outport
  wires:
  Low-Pass Filter (Discrete or Continuous)/1 -> v_e_dot_ref/1
  v_e_ref/1 -> Discrete Derivative/1
  Discrete Derivative/1 -> Low-Pass Filter (Discrete or Continuous)/1

== system Controller/Subsystem/OLD/position_control + autonomous/Guidance/Trajectory Solution Evaluator/Switch Case Action Subsystem1/Map User Input/psi_ref generator ==
  psi_dot : Inport
  yaw_0 : Inport  Port=2
  reset : Inport  Port=3
  Compare To Constant : simulink/Logic and Bit Operations/Compare To Constant  relop=<  const=-2*pi  OutDataTypeStr=boolean
  Compare To Constant1 : simulink/Logic and Bit Operations/Compare To Constant  relop=>=  const=2*pi  OutDataTypeStr=boolean
  Constant : Constant  Value=0
  Delay : Delay  DelayLength=1  InitialConditionSource=Input port  ExternalReset=Rising
      settings: InputPortMap=u0,r5,p4
  Integrator (Discrete or Continuous) : eeGeneralControl/Integrator (Discrete or Continuous)  LabelModeActiveChoice=Discrete  ExternalReset=rising  LimitType=Windup  B=inf  A=-inf  Ts=-1
      settings: LibrarySourceBlock=|
      | ee_sl_lib/General Control/Integrator
      | (Discrete or Continuous)
  Logical Operator : Logic  Operator=OR  Inputs=3  AllPortsSameDT=off  OutDataTypeStr=boolean
  Multiport Switch : MultiPortSwitch  DataPortOrder=Zero-based contiguous  Inputs=2  DiagnosticForDefault=None  zeroidx=on  SaturateOnIntegerOverflow=off  InputSameDT=off
  NOT : Logic  Operator=NOT  IconShape=distinctive  AllPortsSameDT=off  OutDataTypeStr=boolean
  psi : Outport
  wires:
  Multiport Switch/1 -> Integrator (Discrete or Continuous)/3, Delay/3
  NOT/1 -> Multiport Switch/1
  Constant/1 -> Multiport Switch/3
  Delay/1 -> Compare To Constant/1, Compare To Constant1/1
  reset/1 -> Logical Operator/3, Delay/2, NOT/1
  yaw_0/1 -> Multiport Switch/2
  Compare To Constant/1 -> Logical Operator/1
  Compare To Constant1/1 -> Logical Operator/2
  Logical Operator/1 -> Integrator (Discrete or Continuous)/2
  psi_dot/1 -> Integrator (Discrete or Continuous)/1
  Integrator (Discrete or Continuous)/1 -> psi/1, Delay/1  "psi"

== system Controller/Subsystem/OLD/position_control + autonomous/Guidance/Trajectory Solution Evaluator/Switch Case Action Subsystem1/Map User Input/Input Map/Subsystem ==
  Vy_e : Inport
  Vx_e : Inport  Port=2
  States : Inport  Port=3
  Bus Selector1 : BusSelector  OutputSignals=att
  Constant : Constant  Value=0
  Gain : Gain  Gain=-1
  Mux1 : Mux  Inputs=3
  Mux2 : Mux  Inputs=3
  Quaternion Rotation : aerolibutil/Quaternion Rotation
  Rotation Angles to Quaternions : sharedtransform/Rotation Angles to Quaternions  rotationOrder=ZYX  aMode=aMode
  Selector : Selector  InputPortWidth=3  IndexOptions=Index vector (dialog)  Indices=[3]  OutputSizes=1
  Selector1 : Selector  InputPortWidth=3  IndexOptions=Index vector (dialog)  Indices=[1,2]  OutputSizes=1
  "[Vx Vy]_b" : Outport
  wires:
  Gain/1 -> Mux1/1
  Vx_e/1 -> Mux2/1
  Vy_e/1 -> Mux2/2
  Rotation Angles to Quaternions/1 -> Quaternion Rotation/1
  Bus Selector1/1 -> Selector/1  "<att>"
  Selector/1 -> Gain/1
  Quaternion Rotation/1 -> Selector1/1
  Constant/1 -> Mux1/2, Mux1/3, Mux2/3
  Mux2/1 -> Quaternion Rotation/2
  States/1 -> Bus Selector1/1
  Mux1/1 -> Rotation Angles to Quaternions/1
  Selector1/1 -> "[Vx Vy]_b"/1
